simulink model "F16ASYM_Controlled_ACC"  (R2012b)
settings: Solver=ode3  SolverMode=SingleTasking  StartTime=0.0  StopTime=inf  FixedStep=T_sim  RelTol=1e-3
InitFcn:
  | load('NN_c_weights_Last_stable.mat')
values from neighbouring files (symbols this model uses):
  a1 = fitresult.p1    [Stall_protection.m]
  alpha_map_eval = ones(size(M_eval))*NaN    [Auto_trim_aid.m]    (also in Autotrim_maps.mat = [nan nan 0.277598136245 0.119432432992 0.0579479097061 0.027)
  beta_map_eval = ones(size(M_eval))*NaN    [Auto_trim_aid.m]    (also in Autotrim_maps.mat = [nan nan -0.00151549403324 0.00117807579006 -0.0052086799721)
  C_L_0 = fitresult.p2    [Stall_protection.m]
  G_eval = NaN*ones(size(M_sq,2),size(H_sq,2))    [Stall_protection.m]
  H_sq = unique(sort(H_sq))    [Stall_protection.m]
  H_sq_autotrim = min( F_envelope.H_1g):2000:max(F_envelope.H_1g)    [Auto_trim_aid.m]    (also in Autotrim_maps.mat = [0 2000 4000 6000 8000 10000 12000 14000 16000 18000])
  K_b_ACC = params(3)    [Cost_function.m]
  K_b_q = params(4)    [Cost_function.m]
  learning = 20    [Scheduling_desing.m]
  M_sq = unique(sort(M_sq))    [Stall_protection.m]
  M_sq_autotrim = 0:0.1:max(F_envelope.M_1g)    [Auto_trim_aid.m]    (also in Autotrim_maps.mat = [0 0.1 0.2 0.3 0.4 0.5 0.6 0.7 0.8 0.9 1 1.1 ... (21 element)
  Model_used_flag = 1    [Scheduling_desing.m]
  reg_param = 1    [Scheduling_desing.m]
  T_sim = 0.04    [Run_me.m]    (also in Scheduling_desing.m = 0.02)
  tau_ACC = params(1)    [Cost_function.m]
  tau_q = params(2)    [Cost_function.m]
  V_Comp_A_w_z_last = [-0.043311742939 0.0085685727899 -0.0213735657625 0.0330213821126 -0.0306555996667 -0.00573122365227 -0.0106441480787 0.0329440631876 0.0177121952361 -0.0290685435098 -0.0181457235686 -0.0361990502411 ... (1250 elements, 50x25)]    [NN_c_weights_Last_stable.mat]
  V_Comp_last = [-0.0421958473648 0.0184516098779 -0.0436695953504 -0.041154016657 0.00216882652165 -0.0388561228631 0.0327521861474 0.0326079628857 0.0227071838361 -0.0338588476214 0.0161615063846 0.00186003522421 ... (1250 elements, 50x25)]    [NN_c_weights_Last_stable.mat]
  velocity = M_eval(I,J)*a    [Auto_trim_aid.m]    (also in Scheduling_desing.m = M_eval_sche(I,J)*a)
  W_Comp_A_w_z_last = [-0.00689921461652 0.00234704735165 -0.000126421245896 0.00121944724496 6.17702028018e-05 -0.000422762754226 -0.000228913732743 -1.1618795843e-05 7.94007436465e-05 0.000588815786054 2.98617078429e-05 -0.00020420127191 ... (153 elements, 3x51)]    [NN_c_weights_Last_stable.mat]
  W_Comp_last = [-0.00864477030284 0.000183920433695 -0.000300268209456 0.00178165628538 -0.000144806488148 -0.000715209966 -0.000733452792184 5.9552378004e-05 0.000293789747621 0.00184648331608 -0.000150090451416 -0.000741280397229 ... (153 elements, 3x51)]    [NN_c_weights_Last_stable.mat]
undefined symbols (not defined in the file or in its folder): B, DiscIntNeverNeededParam, fi_flag_Simulink, k_B, m_B, sigbuilder_block, Stall_curve, Theta_1_roll_last, Theta_2_roll_last, Theta_3_roll_last, trim_control, trim_state, trim_throttle, V_long_lastA_w_z, V_long_lastAoA, V_roll_last, V_roll_lastMOD, V_yaw_last, W_long_lastA_w_z, W_long_lastAoA, W_roll_last, W_roll_lastMOD, W_yaw_last
libraries: Adaptive_FaultTolerantControl x43, F16_Actuator_Library x14, dspsigops x13, simulink x8, dsparch4 x6, simulink_extras x5, aerolibatmos2 x5, aerolibtransform2 x5, dspmtrx3 x3, qcatlib x2, dspvision x2, dspsnks4 x2
(part 3 of 10)

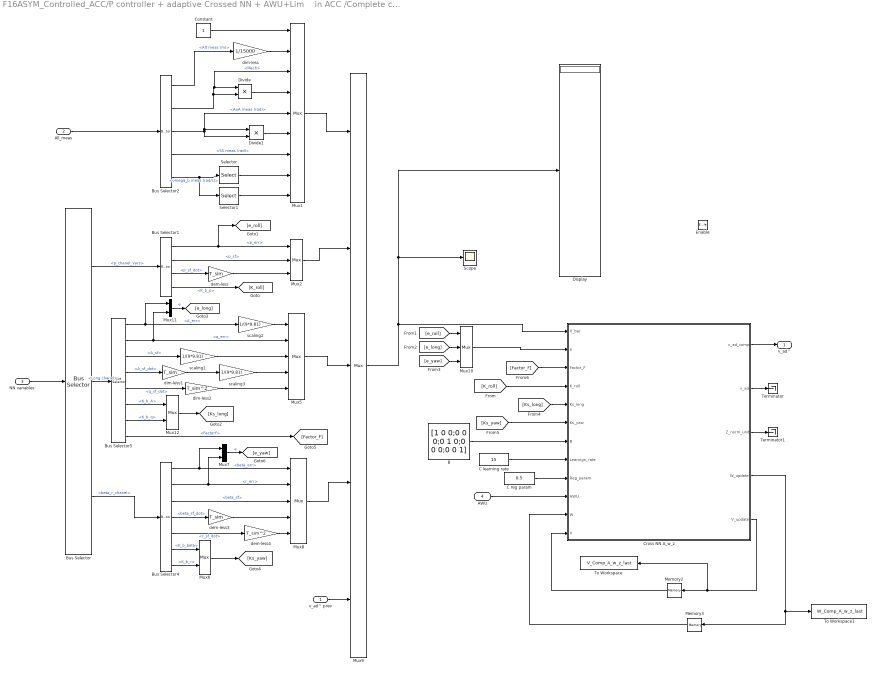
== system F16ASYM_Controlled_ACC/P controller + adaptive Crossed NN + AWU+Lim    in ACC /Complete crossed On-line (adaptive) multi-layer NN: A_w_z ==
  v_ad^ prev : Inport
  All_meas : Inport  Port=2
  NN variables : Inport  Port=3
  AWU : Inport  Port=4
  Enable : EnablePort  StatesWhenEnabling=reset
  B : Constant  Value=[1 0 0;0 0 0;0 1 0;0 0 0;0 0 1]
  Bus Selector : BusSelector  OutputSignals=p_chanel_vars,Long chanel,beta_r_chanel
  Bus Selector1 : BusSelector  OutputSignals=p_err,p_sf,p_sf_dot,K_b_p
  Bus Selector2 : BusSelector  OutputSignals=signal1.Alt meas (m),signal2.Mach,signal1.AoA meas (rad),signal1.SS meas (rad),signal1.omega_b meas (rad/s)
  Bus Selector4 : BusSelector  OutputSignals=beta_chanel vars.beta_err,r_chanel vars.r_err,beta_chanel vars.beta_sf,beta_chanel vars.beta_sf_dot,r_chanel vars.r_sf_dot,beta_chanel vars.K_b_beta,r_chanel vars.K_b_r
  Bus Selector5 : BusSelector  OutputSignals=A_chanel vars.A_err,q_chanel_vars.q_err,A_chanel vars.A_sf,A_chanel vars.A_sf_dot,q_chanel_vars.q_sf_dot,A_chanel vars.K_b_A,q_chanel_vars.K_b_q,A_chanel vars.FactorF
  C learning rate : Constant  Value=15  SampleTime=T_sim
  C reg param : Constant  Value=0.5  SampleTime=T_sim
  Constant : Constant
  Cross NN A_w_z : MATLAB Function  TreatAsAtomicUnit=on
  Display : Display
  Divide : Product  Inputs=**
  Divide1 : Product  Inputs=**
  Memory2 : Memory  X0=V_Comp_A_w_z_last
  Memory3 : Memory  X0=W_Comp_A_w_z_last
  Mux1 : Mux  Inputs=9
  Mux10 : Mux  Inputs=3
  Mux{6..7,11..12} (4 alike) : Mux  Inputs=2
  Mux2 : Mux  Inputs=3
  Mux5 : Mux  Inputs=5
  Mux8 : Mux  Inputs=5
  Mux9 : Mux  Inputs=[9 3 5 5 3]
  Scope : Scope
      settings: SaveName=ScopeData8
  Selector : Selector  InputPortWidth=3  IndexOptions=Index vector (dialog)  Indices=1  OutputSizes=1
  Selector1 : Selector  InputPortWidth=3  IndexOptions=Index vector (dialog)  Indices=3  OutputSizes=1
  Terminator : Terminator
  Terminator1 : Terminator
  To Workspace : ToWorkspace  VariableName=V_Comp_A_w_z_last  SampleTime=-1
      settings: MaxDataPoints=1
  To Workspace1 : ToWorkspace  VariableName=W_Comp_A_w_z_last  SampleTime=-1
      settings: MaxDataPoints=1
  dem-less : Gain  Gain=T_sim
  dem-less3 : Gain  Gain=T_sim
  dem-less4 : Gain  Gain=T_sim^2
  dim-less : Gain  Gain=1/15000
  dim-less1 : Gain  Gain=T_sim
  dim-less2 : Gain  Gain=T_sim^2
  scaling1 : Gain  Gain=1/(9*9.81)
  scaling2 : Gain  Gain=1/(9*9.81)
  scaling3 : Gain  Gain=1/(9*9.81)
  v_ad^ : Outport
  wires:
  [Factor_F] -> Cross NN A_w_z/3(Factor_F)
  Bus Selector5/8 -> [Factor_F]  "<FactorF>"
  scaling3/1 -> Mux5/4
  dim-less2/1 -> Mux5/5
  scaling1/1 -> Mux5/3
  Mux11/1 -> [e_long]  "e"
  Bus Selector/2 -> Bus Selector5/1  "<Long chanel>"
  Bus Selector5/1 -> Mux11/1, scaling2/1  "<A_err>"
  Bus Selector5/2 -> Mux11/2, Mux5/2  "<q_err>"
  Bus Selector5/3 -> scaling1/1  "<A_sf>"
  Bus Selector5/4 -> dim-less1/1  "<A_sf_dot>"
  Bus Selector5/5 -> dim-less2/1  "<q_sf_dot>"
  Bus Selector5/7 -> Mux12/2  "<K_b_q>"
  Bus Selector5/6 -> Mux12/1  "<K_b_A>"
  scaling2/1 -> Mux5/1
  dim-less1/1 -> scaling3/1
  Selector1/1 -> Mux1/9
  [Ks_yaw] -> Cross NN A_w_z/6(Ks_yaw)
  [Ks_long] -> Cross NN A_w_z/5(Ks_long)
  [K_roll] -> Cross NN A_w_z/4(K_roll)
  [e_yaw] -> Mux10/3
  [e_long] -> Mux10/2
  [e_roll] -> Mux10/1
  Mux10/1 -> Cross NN A_w_z/2(e)
  Cross NN A_w_z/4(W_update) -> To Workspace1/1, Memory3/1
  Cross NN A_w_z/5(V_update) -> Memory2/1, To Workspace/1
  Cross NN A_w_z/2(v_ad) -> Terminator/1
  B/1 -> Cross NN A_w_z/7(B)
  Memory3/1 -> Cross NN A_w_z/11(W)
  Memory2/1 -> Cross NN A_w_z/12(V)
  Cross NN A_w_z/1(v_ad_comp) -> v_ad^/1
  C learning rate/1 -> Cross NN A_w_z/8(Learnign_rate)
  C reg param/1 -> Cross NN A_w_z/9(Reg_param)
  Cross NN A_w_z/3(Z_norm_unit) -> Terminator1/1
  Mux9/1 -> Cross NN A_w_z/1(X_bar), Display/1, Scope/1
  v_ad^ prev/1 -> Mux9/5
  Mux8/1 -> Mux9/4
  Mux5/1 -> Mux9/3
  Mux2/1 -> Mux9/2
  Mux1/1 -> Mux9/1
  dem-less4/1 -> Mux8/5
  Mux7/1 -> [e_yaw]  "e"
  Bus Selector4/2 -> Mux7/2, Mux8/2  "<r_err>"
  Bus Selector4/1 -> Mux7/1, Mux8/1  "<beta_err>"
  Mux6/1 -> [Ks_yaw]
  Bus Selector4/6 -> Mux6/1  "<K_b_beta>"
  Bus Selector4/7 -> Mux6/2  "<K_b_r>"
  Bus Selector4/5 -> dem-less4/1  "<r_sf_dot>"
  Bus Selector4/4 -> dem-less3/1  "<beta_sf_dot>"
  Bus Selector4/3 -> Mux8/3  "<beta_sf>"
  dem-less3/1 -> Mux8/4
  Mux12/1 -> [Ks_long]
  dem-less/1 -> Mux2/3
  Bus Selector1/1 -> Mux2/1, [e_roll]  "<p_err>"
  Bus Selector1/2 -> Mux2/2  "<p_sf>"
  Bus Selector1/4 -> [K_roll]  "<K_b_p>"
  Bus Selector2/3 -> Divide1/2, Mux1/5, Divide1/1  "<AoA meas (rad)>"
  Bus Selector2/2 -> Divide/1, Mux1/3, Divide/2  "<Mach>"
  Bus Selector2/4 -> Mux1/7  "<SS meas (rad)>"
  Selector/1 -> Mux1/8
  Bus Selector1/3 -> dem-less/1  "<p_sf_dot>"
  Constant/1 -> Mux1/1
  All_meas/1 -> Bus Selector2/1
  Bus Selector2/1 -> dim-less/1  "<Alt meas (m)>"
  Divide/1 -> Mux1/4
  Divide1/1 -> Mux1/6
  dim-less/1 -> Mux1/2
  Bus Selector2/5 -> Selector/1, Selector1/1  "<omega_b meas (rad/s)>"
  NN variables/1 -> Bus Selector/1
  Bus Selector/1 -> Bus Selector1/1  "<p_chanel_vars>"
  Bus Selector/3 -> Bus Selector4/1  "<beta_r_chanel>"
  AWU/1 -> Cross NN A_w_z/10(AWU)

== system F16ASYM_Controlled_ACC/P controller + adaptive Crossed NN + AWU+Lim    in ACC /Lat_dir Dyn Inversion: beta_dot->r_c ==
  beta_dot_c : Inport
  All_meas : Inport  Port=2
  A_w_y : Selector  InputPortWidth=3  IndexOptions=Index vector (dialog)  Indices=2  OutputSizes=1
  Bus Selector : BusSelector  OutputSignals=signal1.AoA meas (rad),signal1.omega_b meas (rad/s),signal1.V_TAS (m/s),signal2.A_w_CG
  Divide1 : Product  Inputs=**
  Divide3 : Product  Inputs=**
  Divide4 : Product  Inputs=/*
  Divide5 : Product  Inputs=*/
  Selector : Selector  InputPortWidth=3  IndexOptions=Index vector (dialog)  Indices=1  OutputSizes=1
  Trigonometric Function : Trigonometry  Operator=cos
  Trigonometric Function3 : Trigonometry  Operator=tan
  "q_c " : Sum  Inputs=-++
  r_c : Outport
  wires:
  "q_c "/1 -> r_c/1
  Bus Selector/1 -> Trigonometric Function/1, Trigonometric Function3/1  "<AoA meas (rad)>"
  Bus Selector/2 -> Selector/1  "<omega_b meas (rad/s)>"
  Divide1/1 -> "q_c "/2
  Divide3/1 -> Divide4/1
  A_w_y/1 -> Divide4/2
  All_meas/1 -> Bus Selector/1
  Bus Selector/4 -> A_w_y/1  "<A_w_CG>"
  Divide4/1 -> "q_c "/3
  Bus Selector/3 -> Divide3/2  "<V_TAS (m/s)>"
  Trigonometric Function/1 -> Divide3/1, Divide5/2
  Divide5/1 -> "q_c "/1
  beta_dot_c/1 -> Divide5/1
  Trigonometric Function3/1 -> Divide1/1
  Selector/1 -> Divide1/2

== system F16ASYM_Controlled_ACC/P controller + adaptive Crossed NN + AWU+Lim    in ACC /Long Dyn Inversion: alpha_dot ->q ==
  alpha_dot_c : Inport
  All_meas : Inport  Port=2
  Completed : Subsystem
  Manual Switch : ManualSwitch
  Simplified : Subsystem
  q_c : Outport
  wires:
  alpha_dot_c/1 -> Simplified/1(alpha_dot_c), Completed/1(alpha_dot_c)
  All_meas/1 -> Simplified/2(All_meas), Completed/2(All_meas)
  Completed/1(q_c) -> Manual Switch/1
  Simplified/1(q_c) -> Manual Switch/2
  Manual Switch/1 -> q_c/1

== system F16ASYM_Controlled_ACC/P controller + adaptive Crossed NN + AWU+Lim    in ACC /Longitudinal controller in A_w_z ==
  A_w_z des : Inport
  AoA des (rad) : Inport  Port=2
  Anti-windup A_w_z : Inport  Port=3
  Anti-windup AoA : Inport  Port=4
  All meas : Inport  Port=5
  Accel rate --> AoA rate! : Subsystem
  Bus Creator : BusCreator  Inputs=5
  Bus Selector : BusSelector  OutputSignals=signal2.A_w_CG
  Divide : Product  Inputs=**
  Gain : Gain  Gain=-1
  Ref Model and P Controller : Subsystem
  Selector : Selector  InputPortWidth=3  IndexOptions=Index vector (dialog)  Indices=3  OutputSizes=1
  Stall protection : Subsystem  Commented=on
  Sum : Sum  Inputs=+-|
  Terminator : Terminator
  Terminator1 : Terminator
  Terminator2 : Terminator
  A_chanel vars : Outport
  alpha_dot_c : Outport  Port=2
  wires:
  Anti-windup AoA/1 -> Terminator1/1
  AoA des (rad)/1 -> Terminator/1
  Selector/1 -> Gain/1
  Gain/1 -> Ref Model and P Controller/2(y_meas)
  Bus Selector/1 -> Selector/1  "<A_w_CG>"
  Anti-windup A_w_z/1 -> Terminator2/1
  A_w_z des/1 -> Ref Model and P Controller/1(y_ref)
  Ref Model and P Controller/1(y_des_dot) -> Divide/1
  Ref Model and P Controller/2(y_c_ff_dot) -> Bus Creator/1  "A_sf_dot"
  Ref Model and P Controller/3(y_c) -> Bus Creator/2, Sum/1  "A_sf"
  Sum/1 -> Bus Creator/3  "A_err"
  Ref Model and P Controller/4(y_meas_out) -> Sum/2
  Ref Model and P Controller/5(k_b param) -> Bus Creator/4  "K_b_A"
  Bus Creator/1 -> A_chanel vars/1
  Divide/1 -> alpha_dot_c/1
  Accel rate --> AoA rate!/1(A_w  to AoA rates factor) -> Bus Creator/5, Divide/2  "FactorF"
  All meas/1 -> Bus Selector/1, Stall protection/2(All meas), Accel rate --> AoA rate!/1(All_meas)

== system F16ASYM_Controlled_ACC/P controller + adaptive Crossed NN + AWU+Lim    in ACC /Physical limitation ==
  note: Converto to Angular accelerations
  v comm : Inport
  all meas : Inport  Port=2
  Ang Accel : MATLAB Function
  Bus Selector : BusSelector  OutputSignals=signal1.Alt meas (m),signal1.V_TAS (m/s),signal1.AoA meas (rad),signal1.SS meas (rad),signal1.omega_b meas (rad/s),signal1.Throttle_meas
  Bus Selector1 : BusSelector  OutputSignals=signal2.q (Pa),signal1.omega_b meas (rad/s)
  Demux : Demux  Outputs=3
  Display : Display
  Display1 : Display
  Display2 : Display
  Divide : Product  Inputs=**
  Divide1 : Product  Inputs=**
  Gain : Gain  Gain=-1
  Gain1 : Gain
  Mom coefficients that was reached : MATLABFcn  MATLABFcn=Moms_Coeff_estimator  OutputDimensions=3  OutputSignalType=real
  Moments : Subsystem
  Mux : Mux  Inputs=3
  Mux1 : Mux  Inputs=7
  Saturation Dynamic : simulink/Discontinuities/Saturation Dynamic  OutMin=[]  OutMax=[]  OutDataTypeStr=Inherit: Same as second input  OutDataType=fixdt(1, 16)  OutScaling=2^-10  DoSatur=off
  Sign : Signum
  Sign1 : Signum
  max deflections estimator : MATLAB Function  TreatAsAtomicUnit=on
  v limted : Outport
  wires:
  max deflections estimator/1(max_defl) -> Mux1/7
  Mux1/1 -> Mom coefficients that was reached/1
  Bus Selector/5 -> Mux1/5  "<omega_b meas (rad/s)>"
  Bus Selector/1 -> Mux1/1  "<Alt meas (m)>"
  Bus Selector/2 -> Mux1/2  "<V_TAS (m/s)>"
  Bus Selector/3 -> Mux1/3  "<AoA meas (rad)>"
  Bus Selector/4 -> Mux1/4  "<SS meas (rad)>"
  Bus Selector/6 -> Mux1/6  "<Throttle_meas>"
  Ang Accel/2(q_dot) -> Mux/2
  Ang Accel/3(r_dot) -> Mux/3
  Ang Accel/1(p_dot) -> Mux/1
  Bus Selector1/2 -> Ang Accel/4(omega_b)  "<omega_b meas (rad/s)>"
  Moments/3(N) -> Ang Accel/3(N)
  Moments/2(M) -> Ang Accel/2(M)
  Moments/1(L) -> Ang Accel/1(L)
  Bus Selector1/1 -> Moments/4(q)  "<q (Pa)>"
  Demux/3 -> Moments/3(C_N)
  Demux/2 -> Moments/2(C_M)
  Demux/1 -> Moments/1(C_L)
  Mom coefficients that was reached/1 -> Demux/1
  all meas/1 -> Bus Selector/1, Bus Selector1/1
  Mux/1 -> Gain1/1
  v comm/1 -> Saturation Dynamic/2, Display1/1, max deflections estimator/1(v_comm)
  Saturation Dynamic/1 -> Display/1, v limted/1
  Sign/1 -> Divide/1
  Gain1/1 -> Divide/2, Divide1/1, Sign1/1, Display2/1, Sign/1
  Sign1/1 -> Gain/1
  Divide/1 -> Saturation Dynamic/1
  Gain/1 -> Divide1/2
  Divide1/1 -> Saturation Dynamic/3

== system F16ASYM_Controlled_ACC/P controller + adaptive Crossed NN + AWU+Lim    in ACC /Sigmoid  ==
  In : Inport
  Display : Display
  Fcn1 : Fcn  Commented=on  Expr=2.0 ./ (1.0 + exp(-u(4)*u(1:3)))-1
  MATLAB Function : MATLAB Function  TreatAsAtomicUnit=on
  a : Constant  Value=a
  Out : Outport
  wires:
  MATLAB Function/1(y) -> Display/1, Out/1
  In/1 -> MATLAB Function/1(u)
  a/1 -> MATLAB Function/2(a)

== matlab function F16ASYM_Controlled_ACC/Primary Controller/P controller + adaptive Isolated NN/On-line (adaptive) multi-layer NNs SIMPL/Roll NN/Roll 2HL NN/Roll Multilayer NN ==
  data: X_bar input size=[12,1]; v_ad_comp output; e input size=1; P input; B input; Roll_learnign_rate input size=1; Roll_reg_param input size=1; Theta_1 input size=[30,12]; Theta_2 input size=[20,31]; Theta_3 input size=[1,21]; v_ad output; Z_norm_unit output; T_sim parameter; Theta_1_update output; Theta_2_update output; Theta_3_update output
function [v_ad_comp,v_ad,Z_norm_unit,Theta_1_update,Theta_2_update,Theta_3_update]  = Roll_ML_NN(X_bar,e,P,B,Roll_learnign_rate, Roll_reg_param,Theta_1,Theta_2,Theta_3,T_sim)

%% Compute prelimiary parameters
zeta= e'*P*B;

%% Feedforward. Layers: Sigmoidal, linear, linear

a2=[1 ;  sigmoid( Theta_1*X_bar )]; % Sigmoidal
a3=[1 ;  (Theta_2*a2)]; % Linear
% z4=Theta_3*a3;
% a4 = z4; % Linear
% v_ad =a4;

% Backward
% % delta4=zeta; % In this particular case of adaptive NN, this error is a weighted tracking error
delta3=Theta_3'*zeta;
delta2=Theta_2'*delta3(2:end).*(a2.*(ones(size(a2))-a2)); 


%% Compute the gradients or adaptation laws
Gamma_Theta_3= Roll_learnign_rate; %  learnign rate
Gamma_Theta_2 = Roll_learnign_rate; % learning rate
Gamma_Theta_1= Roll_learnign_rate; % learning rate
lambda = Roll_reg_param;    % Regularization constant

% % Theta_1_dot=zeros(size(Theta_1));
% % Theta_2_dot=zeros(size(Theta_2));
% % Theta_3_dot=zeros(size(Theta_3));

Theta_3_dot = -Gamma_Theta_3*zeta*a3' ;
Theta_3_dot(:,2:end) =  Theta_3_dot(:,2:end) - Gamma_Theta_3*lambda*norm(zeta).*Theta_3(:,2:end);

Theta_2_dot= -Gamma_Theta_2*( delta3(2:end)*a2'   + lambda*norm(zeta).*Theta_2);
Theta_2_dot(:,2:end) =  Theta_2_dot(:,2:end) - Gamma_Theta_2*lambda*norm(zeta).*Theta_2(:,2:end);

Theta_1_dot= -Gamma_Theta_1*( delta2(2:end)*X_bar'   + lambda*norm(zeta).*Theta_1);
Theta_1_dot(:,2:end) =  Theta_1_dot(:,2:end) - Gamma_Theta_1*lambda*norm(zeta).*Theta_1(:,2:end);


%% Adaptation
Theta_1_update = Theta_1 + T_sim*Theta_1_dot;
Theta_2_update = Theta_2 + T_sim*Theta_2_dot;
Theta_3_update = Theta_3 + T_sim*Theta_3_dot;

%% re-compute v_ad

a2=[1 ;  sigmoid( Theta_1_update*X_bar )]; % Sigmoidal
a3=[1 ;  (Theta_2_update*a2)]; % Linear
v_ad=Theta_3_update*a3;


%% Compute v_ad_comp
% Z = blkdiag( Theta_1_update , Theta_2_update , Theta_3_update );

Z =  [ Theta_1_update, zeros(size(Theta_1_update,1),size(Theta_2_update,2)) , zeros(size(Theta_1_update,1),size(Theta_3_update,2));
            zeros(size(Theta_2_update,1),size(Theta_1_update,2)) , Theta_2_update , zeros(size(Theta_2_update,1),size(Theta_3_update,2)) ;
            zeros(size(Theta_3_update,1),size(Theta_1_update,2)),zeros(size(Theta_3_update,1),size(Theta_2_update,2)),  Theta_3_update ];

Z_norm = norm(Z,'fro');
Z_max = min(size(Theta_1))*min(size(Theta_2))*min(size(Theta_3));
Z_norm_unit = Z_norm;

K_r0= 0.02;
K_r1= 0;
v_r0 = -K_r0*zeta;
v_r1 = -K_r1*(Z_norm+Z_max)*zeta;

v_ad_comp = v_ad + v_r1 +v_r0;


end

== matlab function F16ASYM_Controlled_ACC/Control allocator/Control allocator: NO RECONF/MATLAB Function ==
  data: Deflections input; Saturations output; Sup_lim input; Inf_lim input
function Saturations = Saturations(Deflections,Sup_lim,Inf_lim)
Saturations=zeros(7,1);

for i=1:7
    
    if Deflections(i)>=Sup_lim(i)
        Saturations(i)=1;
    elseif Deflections(i)<=Inf_lim(i)
        Saturations(i)=-1;
    else
        Saturations(i)=0;
    end
end

== matlab function F16ASYM_Controlled_ACC/Anti-windup Calculation/Anti-windup: Reconfigurable/Antiwindup calculation ==
  data: Ang_acell_comm input; AWU output; Ang_acell_achieved input; Saturations input; B input; deflections input
function AWU = AWU_calculation(Ang_acell_comm,Ang_acell_achieved,Saturations,B,deflections)
% Computing Saturation limits
sup_limit = [24,24,21,21,29,25,25]-1;
inf_limit = [-24,-24,-21,-21,-29,0,0]+1;

for i=1:7
    Saturations(i) = Saturation_smooth(abs(Saturations(i)),deflections(i),sup_limit(i),inf_limit(i));
end
Sat_B = B*Saturations;
B_max = B*ones(7,1);

AWU=zeros(3,1);

%% Method A
% % psi = 0.01; % % of the effort above the one we consider manouvreability is reduced
% % for i=1:3
% %     if i==1 && sign(deflections(3))== sign(deflections(4)) && abs(Sat_B(i))>psi*abs(B_max(i))
% %         AWU(2) = Ang_acell_comm(2) - Ang_acell_achieved(2); % we have to desaturate longitudinally not laterally
% %     elseif  i==1 && sign(deflections(3))~= sign(deflections(4)) && abs(Sat_B(i))>psi*abs(B_max(i))
% %         AWU(i) = Ang_acell_comm(i) - Ang_acell_achieved(i);
% %     elseif i~=1 && abs(Sat_B(i))>psi*abs(B_max(i))
% %         AWU(i) = Ang_acell_comm(i) - Ang_acell_achieved(i);
% %     end 
% % end

%% Method B
% % % Long
% % if Saturations(1)~=0 || Saturations(2)~=0 ||  Saturations(6)~=0 || Saturations(7)~=0 || ((Saturations(3)~=0 || Saturations(4)~=0) && sign(deflections(3))== sign(deflections(4)) ) 
% %     AWU(2) = Ang_acell_comm(2) - Ang_acell_achieved(2);
% % end
% % % Lat-dir
% % if ((Saturations(3)~=0 || Saturations(4)~=0) && sign(deflections(3)) ~= sign(deflections(4)) )  || Saturations(5)~=0 || Saturations(6)~=0 || Saturations(7)~=0
% %     AWU(1) = Ang_acell_comm(1) - Ang_acell_achieved(1);
% %     AWU(3) = Ang_acell_comm(3) - Ang_acell_achieved(3);
% % 
% % end


%% Method C
for i=1:3
        AWU(i) = (Ang_acell_comm(i) - Ang_acell_achieved(i))*Sat_B(i)/norm(B(i,:));
end

end

function Saturation_out = Saturation_smooth(Saturation,angle,sup_limit,inf_limit)

a=5;
Saturation_out  = ( 1 - 1./(1+exp(-a*(angle-inf_limit ))) + 1./(1+exp(-a*(angle-sup_limit ))) )*Saturation;


end

== matlab function F16ASYM_Controlled_ACC/Primary Controller/P  + Crossed NN + AWU+Lim + hand-over/P controller + adaptive Crossed NN + AWU+Lim   in AoA/Physical limitation/Ang Accel ==
  data: L input; p_dot output; q_dot output; r_dot output; M input; N input; omega_b input
function [p_dot,q_dot,r_dot] = Ang_accel(L,M,N,omega_b)
Jy  = 75673.6;
Jxz = 1331.4; 
Jz  = 85552.1;  
Jx  = 12874.8;
h_E = 216.9;

denom = Jx*Jz - Jxz*Jxz;

% % C1 = ((Jy - Jz)  * Jz  - (Jxz * Jxz))/ Gamma;
% % C2 = ((Jx - Jy + Jz ) * Jxz ) / Gamma;
% % C3 = Jz / Gamma;
% % C4 = Jxz / Gamma;
% % C5 = (Jz - Jx) / Jy;
% % C6 = Jxz / Jy ;
% % C7 = 1 / Jy;
% % C8 = (Jx * (Jx - Jy ) + Jxz * Jxz) / Gamma;
% % C9 = Jx / Gamma;


p_dot =  (Jz*L + Jxz*N - (Jz*(Jz-Jy)+Jxz*Jxz)*omega_b(2)*omega_b(3) + Jxz*(Jx-Jy+Jz)*omega_b(1)*omega_b(2) + Jxz*omega_b(2)*h_E)/denom;

q_dot = (M + (Jz-Jx)*omega_b(1)*omega_b(3) - Jxz*(omega_b(1)*omega_b(1)-omega_b(3)*omega_b(3)) - omega_b(3)*h_E)/Jy;


r_dot = (Jx*N + Jxz*L + (Jx*(Jx-Jy)+Jxz*Jxz)*omega_b(1)*omega_b(2) - Jxz*(Jx-Jy+Jz)*omega_b(2)*omega_b(3) +  Jx*omega_b(2)*h_E)/denom;

== matlab function F16ASYM_Controlled_ACC/P controller + adaptive Crossed NN + AWU+Lim    in ACC /Physical limitation/Ang Accel ==
  data: L input; p_dot output; q_dot output; r_dot output; M input; N input; omega_b input
function [p_dot,q_dot,r_dot] = Ang_accel(L,M,N,omega_b)
Jy  = 75673.6;
Jxz = 1331.4; 
Jz  = 85552.1;  
Jx  = 12874.8;
h_E = 216.9;

denom = Jx*Jz - Jxz*Jxz;

% % C1 = ((Jy - Jz)  * Jz  - (Jxz * Jxz))/ Gamma;
% % C2 = ((Jx - Jy + Jz ) * Jxz ) / Gamma;
% % C3 = Jz / Gamma;
% % C4 = Jxz / Gamma;
% % C5 = (Jz - Jx) / Jy;
% % C6 = Jxz / Jy ;
% % C7 = 1 / Jy;
% % C8 = (Jx * (Jx - Jy ) + Jxz * Jxz) / Gamma;
% % C9 = Jx / Gamma;


p_dot =  (Jz*L + Jxz*N - (Jz*(Jz-Jy)+Jxz*Jxz)*omega_b(2)*omega_b(3) + Jxz*(Jx-Jy+Jz)*omega_b(1)*omega_b(2) + Jxz*omega_b(2)*h_E)/denom;

q_dot = (M + (Jz-Jx)*omega_b(1)*omega_b(3) - Jxz*(omega_b(1)*omega_b(1)-omega_b(3)*omega_b(3)) - omega_b(3)*h_E)/Jy;


r_dot = (Jx*N + Jxz*L + (Jx*(Jx-Jy)+Jxz*Jxz)*omega_b(1)*omega_b(2) - Jxz*(Jx-Jy+Jz)*omega_b(2)*omega_b(3) +  Jx*omega_b(2)*h_E)/denom;

== system F16ASYM_Controlled_ACC/Primary Controller/P  + Crossed NN + AWU+Lim + hand-over ==
  note: Indicator correspond to 1
  note: Indicator correspond to 0
  A_w_z des : Inport
  AoA des (rad) : Inport  Port=2
  p des (rad/s) : Inport  Port=3
  beta des (rad) : Inport  Port=4
  Anti-windup A_w_z : Inport  Port=5
  Anti-windup AoA : Inport  Port=6
  Anti-windup beta : Inport  Port=7
  All measures : Inport  Port=8
  Anti-windup signals : Inport  Port=9
  A_w_z des1 : InportShadow
  Anti-windup A_w_z1 : InportShadow  Port=5
  Anti-windup AoA1 : InportShadow  Port=6
  Anti-windup beta1 : InportShadow  Port=7
  Anti-windup signals1 : InportShadow  Port=9
  AoA des (rad)1 : InportShadow  Port=2
  Bus Selector : BusSelector  OutputSignals=signal2.a,signal1.V_TAS (m/s)
  Gain2 : Gain  Gain=2
  Logical Operator : Logic  Operator=NOT  AllPortsSameDT=off  OutDataTypeStr=boolean
  Min TAS : Product  Inputs=**
  "P controller + adaptive Crossed NN + AWU+Lim    in ACC " : Subsystem  VariantObject=Adaptive Controller Crossed+AWU+Lim
  P controller + adaptive Crossed NN + AWU+Lim   in AoA : Subsystem  VariantObject=Adaptive Controller Crossed+AWU+Lim
  Relational Operator5 : RelationalOperator  OutDataTypeStr=boolean
  Scope : Scope
      settings: YMin=-2.75  YMax=0.25  SaveName=ScopeData32
  Scope1 : Scope  Commented=on
      settings: YMin=-2.75  YMax=0.25  SaveName=ScopeData33
  Switch : Switch  Commented=on  Threshold=0.5  InputSameDT=on
  Transition smoother : MATLAB Function  Commented=on  TreatAsAtomicUnit=on
  "Transitions Smotother " : Subsystem
  Transitions Smotother 1 : Subsystem  Commented=on
  Unit Delay : UnitDelay  Commented=on  SampleTime=-1
  beta des (rad)1 : InportShadow  Port=4
  p des (rad/s)1 : InportShadow  Port=3
  Angular acc des : Outport
  Control_in : Outport  Port=2
  wires:
  Anti-windup signals/1 -> P controller + adaptive Crossed NN + AWU+Lim   in AoA/9(Anti-windup signals)
  Anti-windup beta/1 -> P controller + adaptive Crossed NN + AWU+Lim   in AoA/7(Anti-windup beta)
  A_w_z des/1 -> P controller + adaptive Crossed NN + AWU+Lim   in AoA/1(A_w_z des)
  Anti-windup A_w_z/1 -> P controller + adaptive Crossed NN + AWU+Lim   in AoA/5(Anti-windup A_w_z)
  Anti-windup AoA/1 -> P controller + adaptive Crossed NN + AWU+Lim   in AoA/6(Anti-windup AoA)
  AoA des (rad)/1 -> P controller + adaptive Crossed NN + AWU+Lim   in AoA/2(AoA des (rad))
  beta des (rad)/1 -> P controller + adaptive Crossed NN + AWU+Lim   in AoA/4(beta des (rad))
  p des (rad/s)/1 -> P controller + adaptive Crossed NN + AWU+Lim   in AoA/3(p des (rad/s))
  A_w_z des1/1 -> "P controller + adaptive Crossed NN + AWU+Lim    in ACC "/1(A_w_z des)
  AoA des (rad)1/1 -> "P controller + adaptive Crossed NN + AWU+Lim    in ACC "/2(AoA des (rad))
  p des (rad/s)1/1 -> "P controller + adaptive Crossed NN + AWU+Lim    in ACC "/3(p des (rad/s))
  beta des (rad)1/1 -> "P controller + adaptive Crossed NN + AWU+Lim    in ACC "/4(beta des (rad))
  Anti-windup A_w_z1/1 -> "P controller + adaptive Crossed NN + AWU+Lim    in ACC "/5(Anti-windup A_w_z)
  Anti-windup AoA1/1 -> "P controller + adaptive Crossed NN + AWU+Lim    in ACC "/6(Anti-windup AoA)
  Anti-windup beta1/1 -> "P controller + adaptive Crossed NN + AWU+Lim    in ACC "/7(Anti-windup beta)
  All measures/1 -> "P controller + adaptive Crossed NN + AWU+Lim    in ACC "/8(All measures), Bus Selector/1, P controller + adaptive Crossed NN + AWU+Lim   in AoA/8(All measures)
  Anti-windup signals1/1 -> "P controller + adaptive Crossed NN + AWU+Lim    in ACC "/9(Anti-windup signals)
  [Min_Mach] -> Min TAS/1  "Min M"
  Bus Selector/1 -> Min TAS/2  "<a>"
  Min TAS/1 -> Gain2/1
  Gain2/1 -> Relational Operator5/1
  Bus Selector/2 -> Relational Operator5/2  "<V_TAS (m/s)>"
  "P controller + adaptive Crossed NN + AWU+Lim    in ACC "/1(Angular acc des) -> "Transitions Smotother "/3(From  ACC)
  P controller + adaptive Crossed NN + AWU+Lim   in AoA/1(Angular acc des) -> "Transitions Smotother "/1(From AoA)
  Relational Operator5/1 -> Logical Operator/1, Control_in/1, "Transitions Smotother "/2(Indicator), P controller + adaptive Crossed NN + AWU+Lim   in AoA/10(Active)
  Transition smoother/2(indicator_out) -> Unit Delay/1
  Unit Delay/1 -> Transition smoother/4(indicator_prev)
  "Transitions Smotother "/1(Ang accels comm) -> Angular acc des/1, Scope/1
  Switch/1 -> Scope1/1
  Logical Operator/1 -> "P controller + adaptive Crossed NN + AWU+Lim    in ACC "/10(Active)

== system F16ASYM_Controlled_ACC/Primary Controller/P controller ==
  A_w_z des : Inport
  AoA des (rad) : Inport  Port=2
  p des (rad/s) : Inport  Port=3
  beta des (rad) : Inport  Port=4
  Anti-windup A_w_z : Inport  Port=5
  Anti-windup AoA : Inport  Port=6
  Anti-windup beta : Inport  Port=7
  All measures : Inport  Port=8
  Anti-windup signals : Inport  Port=9
  Body Rates Controller : Subsystem
  Bus Creator2 : BusCreator
  Bus Selector3 : BusSelector  OutputSignals=signal1.SS meas (rad)
  Constant : Constant  Value=NaN
  Display : Display
  Display1 : Display
  Lat_dir Dyn Inversion: beta_dot->r_c : Subsystem
  Long Dyn Inversion: alpha_dot ->q : Subsystem
  Longitudinal Controller: AoA or A_w_z : Subsystem  Variant=on  OverrideUsingVariant=Controller of AoA
  Ref Model and P Controller : Adaptive_FaultTolerantControl/Ref Model and P Controller  tau=0.4  y_i=trim_state(9)  K_f=1  K_b=5
  Sum1 : Sum  Inputs=+-|
  Terminator : Terminator
  Terminator1 : Terminator
  Terminator2 : Terminator
  Angular acc des : Outport
  Control_in : Outport  Port=2
  wires:
  Anti-windup beta/1 -> Terminator1/1
  Ref Model and P Controller/5 -> Bus Creator2/4  "K_b_beta"
  Ref Model and P Controller/4 -> Sum1/2
  Sum1/1 -> Bus Creator2/3  "beta_err"
  Ref Model and P Controller/3 -> Bus Creator2/2, Sum1/1  "beta_sf"
  Ref Model and P Controller/2 -> Bus Creator2/1  "beta_sf_dot"
  Anti-windup signals/1 -> Terminator/1
  All measures/1 -> Longitudinal Controller: AoA or A_w_z/5(All meas), Long Dyn Inversion: alpha_dot ->q/2(All_meas), Bus Selector3/1, Lat_dir Dyn Inversion: beta_dot->r_c/2(All_meas), Body Rates Controller/4(All_meas)
  A_w_z des/1 -> Longitudinal Controller: AoA or A_w_z/1(A_w_z des)
  Anti-windup A_w_z/1 -> Longitudinal Controller: AoA or A_w_z/3(Anti-windup A_w_z)
  Anti-windup AoA/1 -> Longitudinal Controller: AoA or A_w_z/4(Anti-windup AoA)
  AoA des (rad)/1 -> Longitudinal Controller: AoA or A_w_z/2(AoA des (rad))
  Longitudinal Controller: AoA or A_w_z/3(alpha_dot_c) -> Display/1, Long Dyn Inversion: alpha_dot ->q/1(alpha_dot_c)
  beta des (rad)/1 -> Ref Model and P Controller/1
  Long Dyn Inversion: alpha_dot ->q/1(q_c) -> Body Rates Controller/2(q_ref), Display1/1
  p des (rad/s)/1 -> Body Rates Controller/1(p_ref)
  Ref Model and P Controller/1 -> Lat_dir Dyn Inversion: beta_dot->r_c/1(beta_dot_c)
  Bus Selector3/1 -> Ref Model and P Controller/2  "<SS meas (rad)>"
  Lat_dir Dyn Inversion: beta_dot->r_c/1(r_c) -> Body Rates Controller/3(r_ref)
  Bus Creator2/1 -> Terminator2/1  "beta_chanel vars"
  Body Rates Controller/1(Angular acc des (rad/s^2)) -> Angular acc des/1  "v_p+v_dot_ff"
  Constant/1 -> Control_in/1

== system F16ASYM_Controlled_ACC/Primary Controller/P controller + adaptive Crossed NN ==
  A_w_z des : Inport
  AoA des (rad) : Inport  Port=2
  p des (rad/s) : Inport  Port=3
  beta des (rad) : Inport  Port=4
  Anti-windup A_w_z : Inport  Port=5
  Anti-windup AoA : Inport  Port=6
  Anti-windup beta : Inport  Port=7
  All measures : Inport  Port=8
  Anti-windup signals : Inport  Port=9
  Body Rates Controller : Subsystem
  Bus Creator : BusCreator  Inputs=3
  Bus Creator1 : BusCreator  Inputs=3
  Bus Creator2 : BusCreator
  Bus Creator3 : BusCreator  Inputs=2
  Bus Selector3 : BusSelector  OutputSignals=signal1.SS meas (rad)
  Complete crossed On-line (adaptive) multi-layer NN : Subsystem  Variant=on  OverrideUsingVariant=NN on A_w_z
      mask Display:
      | image(imread('ANN.png'))
      | 
      | port_label('input', 1, 'v prev')
      | port_label('input', 2, 'All meas')
      | port_label('input', 3, 'NN vars')
      | 
      | port_label('output', 1, 'v_ad^')
  Display{,1..6} (7 alike) : Display
  Ground : Ground
  Lat_dir Dyn Inversion: beta_dot->r_c : Subsystem
  Long Dyn Inversion: alpha_dot ->q : Subsystem
  Longitudinal Controller: AoA or A_w_z : Subsystem  Variant=on  OverrideUsingVariant=Controller of A_w_z
  Memory : Memory  X0=[0,0,0]
  Ref Model and P Controller : Adaptive_FaultTolerantControl/Ref Model and P Controller  tau=0.45  y_i=trim_state(9)  K_f=1  K_b=5
  "Sigmoid " : Subsystem  mask{a=0.15}
      mask prompts: a "Sigmoid a param"
      mask TypeOptions a: a/Value
      mask Display:
      | x=-25:0.1:25;
      | 
      | y=(2.0 ./ (1.0 + exp(-a.*x))-1) ;
      | y2=zeros(size(x));
      | 
      | plot(x,y,x,y2);
      | 
      | text(-12,0.5, ['a= ',num2str(a)])
  Sum : Sum  Inputs=-+|
  Sum1 : Sum  Inputs=+-|
  Terminator : Terminator
  Terminator1 : Terminator
  Angular acc des : Outport
  Control_in : Outport  Port=2
  wires:
  Anti-windup signals/1 -> Terminator/1
  Ref Model and P Controller/1 -> Lat_dir Dyn Inversion: beta_dot->r_c/1(beta_dot_c), Display5/1
  Complete crossed On-line (adaptive) multi-layer NN/1(v_ad^) -> Display2/1, Sum/1  "v_ad^"
  "Sigmoid "/1(Out) -> Memory/1
  Anti-windup beta/1 -> Terminator1/1
  Bus Creator3/1 -> Bus Creator/3  "beta_r_chanel"
  Bus Creator2/1 -> Bus Creator3/2  "beta_chanel vars"
  Body Rates Controller/3(r_chanel vars) -> Bus Creator3/1  "r_chanel vars"
  Ref Model and P Controller/5 -> Bus Creator2/4  "K_b_beta"
  Ref Model and P Controller/4 -> Sum1/2
  Sum1/1 -> Bus Creator2/3  "beta_err"
  Ref Model and P Controller/3 -> Bus Creator2/2, Sum1/1  "beta_sf"
  Ref Model and P Controller/2 -> Bus Creator2/1  "beta_sf_dot"
  Bus Creator1/1 -> Bus Creator/1  "Long chanel"
  Longitudinal Controller: AoA or A_w_z/2(alpha_chanel vars) -> Bus Creator1/2  "alpha_chanel vars"
  Longitudinal Controller: AoA or A_w_z/1(A_chanel vars) -> Bus Creator1/1  "A_chanel vars"
  Body Rates Controller/1(q_chanel vars) -> Bus Creator1/3  "q_chanel_vars"
  Body Rates Controller/2(p_chanel vars) -> Bus Creator/2  "p_chanel_vars"
  Memory/1 -> Complete crossed On-line (adaptive) multi-layer NN/1(v_ad^ prev)
  Bus Creator/1 -> Complete crossed On-line (adaptive) multi-layer NN/3(NN variables)
  Body Rates Controller/4(Angular acc des (rad/s^2)) -> Sum/2, Display3/1  "v_p+v_dot_ff"
  All measures/1 -> Longitudinal Controller: AoA or A_w_z/5(All meas), Long Dyn Inversion: alpha_dot ->q/2(All_meas), Bus Selector3/1, Lat_dir Dyn Inversion: beta_dot->r_c/2(All_meas), Body Rates Controller/4(All_meas), Complete crossed On-line (adaptive) multi-layer NN/2(All_meas)
  Sum/1 -> Angular acc des/1, "Sigmoid "/1(In), Display4/1  "v"
  A_w_z des/1 -> Longitudinal Controller: AoA or A_w_z/1(A_w_z des)
  Anti-windup A_w_z/1 -> Longitudinal Controller: AoA or A_w_z/3(Anti-windup A_w_z)
  Anti-windup AoA/1 -> Longitudinal Controller: AoA or A_w_z/4(Anti-windup AoA)
  AoA des (rad)/1 -> Longitudinal Controller: AoA or A_w_z/2(AoA des (rad))
  Longitudinal Controller: AoA or A_w_z/3(alpha_dot_c) -> Display/1, Long Dyn Inversion: alpha_dot ->q/1(alpha_dot_c)
  beta des (rad)/1 -> Ref Model and P Controller/1
  Long Dyn Inversion: alpha_dot ->q/1(q_c) -> Body Rates Controller/2(q_ref), Display1/1
  p des (rad/s)/1 -> Body Rates Controller/1(p_ref)
  Bus Selector3/1 -> Ref Model and P Controller/2  "<SS meas (rad)>"
  Lat_dir Dyn Inversion: beta_dot->r_c/1(r_c) -> Body Rates Controller/3(r_ref), Display6/1
  Ground/1 -> Control_in/1

== system F16ASYM_Controlled_ACC/Primary Controller/P controller + adaptive Crossed NN + AWU+Lim  ==
  A_w_z des : Inport
  AoA des (rad) : Inport  Port=2
  p des (rad/s) : Inport  Port=3
  beta des (rad) : Inport  Port=4
  Anti-windup A_w_z : Inport  Port=5
  Anti-windup AoA : Inport  Port=6
  Anti-windup beta : Inport  Port=7
  All measures : Inport  Port=8
  Anti-windup signals : Inport  Port=9
  Body Rates Controller : Subsystem
  Bus Creator : BusCreator  Inputs=3
  Bus Creator1 : BusCreator  Inputs=3
  Bus Creator2 : BusCreator
  Bus Creator3 : BusCreator  Inputs=2
  Bus Selector3 : BusSelector  OutputSignals=signal1.SS meas (rad)
  Complete crossed On-line (adaptive) multi-layer NN : Subsystem  Variant=on  OverrideUsingVariant=NN on AoA
      mask Display:
      | image(imread('ANN.png'))
      | 
      | port_label('input', 1, 'v prev')
      | port_label('input', 2, 'All meas')
      | port_label('input', 3, 'NN vars')
      | port_label('input', 4, 'Anti-windup')
      | 
      | port_label('output', 1, 'v_ad^')
  Constant : Constant  Value=NaN
  Display{,1..3,5..6} (6 alike) : Display
  "Display4 " : Display
  Lat_dir Dyn Inversion: beta_dot->r_c : Subsystem
  Long Dyn Inversion: alpha_dot ->q : Subsystem
  Longitudinal Controller: AoA or A_w_z : Subsystem  Variant=on  OverrideUsingVariant=Controller of AoA
  Memory : Memory  X0=[0,0,0]
  Physical limitation : Subsystem
  Ref Model and P Controller : Adaptive_FaultTolerantControl/Ref Model and P Controller  tau=0.45  y_i=trim_state(9)  K_f=1  K_b=5
  Scope1 : Scope
      settings: YMin=-8000  YMax=9000  SaveName=ScopeData27
  "Sigmoid " : Subsystem  mask{a=0.15}
      mask prompts: a "Sigmoid a param"
      mask TypeOptions a: a/Value
      mask Display:
      | x=-25:0.1:25;
      | 
      | y=(2.0 ./ (1.0 + exp(-a.*x))-1) ;
      | y2=zeros(size(x));
      | 
      | plot(x,y,x,y2);
      | 
      | text(-12,0.5, ['a= ',num2str(a)])
  Sum : Sum  Inputs=-+|
  Sum1 : Sum  Inputs=+-|
  Terminator1 : Terminator
  Angular acc des : Outport
  Control_in : Outport  Port=2
  wires:
  Lat_dir Dyn Inversion: beta_dot->r_c/1(r_c) -> Display6/1, Body Rates Controller/3(r_ref)
  Bus Selector3/1 -> Ref Model and P Controller/2  "<SS meas (rad)>"
  p des (rad/s)/1 -> Body Rates Controller/1(p_ref)
  Long Dyn Inversion: alpha_dot ->q/1(q_c) -> Body Rates Controller/2(q_ref), Display1/1
  beta des (rad)/1 -> Ref Model and P Controller/1
  Longitudinal Controller: AoA or A_w_z/3(alpha_dot_c) -> Long Dyn Inversion: alpha_dot ->q/1(alpha_dot_c), Display/1
  AoA des (rad)/1 -> Longitudinal Controller: AoA or A_w_z/2(AoA des (rad))
  Anti-windup AoA/1 -> Longitudinal Controller: AoA or A_w_z/4(Anti-windup AoA)
  Anti-windup A_w_z/1 -> Longitudinal Controller: AoA or A_w_z/3(Anti-windup A_w_z)
  A_w_z des/1 -> Longitudinal Controller: AoA or A_w_z/1(A_w_z des)
  Sum/1 -> "Display4 "/1, "Sigmoid "/1(In), Physical limitation/1(v comm)  "v"
  All measures/1 -> Complete crossed On-line (adaptive) multi-layer NN/2(All_meas), Physical limitation/2(all meas), Body Rates Controller/4(All_meas), Lat_dir Dyn Inversion: beta_dot->r_c/2(All_meas), Bus Selector3/1, Long Dyn Inversion: alpha_dot ->q/2(All_meas), Longitudinal Controller: AoA or A_w_z/5(All meas)
  Body Rates Controller/4(Angular acc des (rad/s^2)) -> Display3/1, Sum/2  "v_p+v_dot_ff"
  Bus Creator/1 -> Complete crossed On-line (adaptive) multi-layer NN/3(NN variables)
  Memory/1 -> Complete crossed On-line (adaptive) multi-layer NN/1(v_ad^ prev)
  Body Rates Controller/2(p_chanel vars) -> Bus Creator/2  "p_chanel_vars"
  Body Rates Controller/1(q_chanel vars) -> Bus Creator1/3  "q_chanel_vars"
  Longitudinal Controller: AoA or A_w_z/1(A_chanel vars) -> Bus Creator1/1  "A_chanel vars"
  Longitudinal Controller: AoA or A_w_z/2(alpha_chanel vars) -> Bus Creator1/2  "alpha_chanel vars"
  Bus Creator1/1 -> Bus Creator/1  "Long chanel"
  Ref Model and P Controller/2 -> Bus Creator2/1  "beta_sf_dot"
  Ref Model and P Controller/3 -> Sum1/1, Bus Creator2/2  "beta_sf"
  Sum1/1 -> Bus Creator2/3  "beta_err"
  Ref Model and P Controller/4 -> Sum1/2
  Ref Model and P Controller/5 -> Bus Creator2/4  "K_b_beta"
  Body Rates Controller/3(r_chanel vars) -> Bus Creator3/1  "r_chanel vars"
  Bus Creator2/1 -> Bus Creator3/2  "beta_chanel vars"
  Bus Creator3/1 -> Bus Creator/3  "beta_r_chanel"
  Anti-windup beta/1 -> Terminator1/1
  "Sigmoid "/1(Out) -> Memory/1
  Complete crossed On-line (adaptive) multi-layer NN/1(v_ad^) -> Scope1/1, Display2/1, Sum/1  "v_ad^"
  Ref Model and P Controller/1 -> Display5/1, Lat_dir Dyn Inversion: beta_dot->r_c/1(beta_dot_c)
  Anti-windup signals/1 -> Complete crossed On-line (adaptive) multi-layer NN/4(AWU)
  Physical limitation/1(v limted) -> Angular acc des/1
  Constant/1 -> Control_in/1

== system F16ASYM_Controlled_ACC/Primary Controller/P controller + adaptive Isolated NN ==
  A_w_z des : Inport
  AoA des (rad) : Inport  Port=2
  p des (rad/s) : Inport  Port=3
  beta des (rad) : Inport  Port=4
  Anti-windup A_w_z : Inport  Port=5
  Anti-windup AoA : Inport  Port=6
  Anti-windup beta : Inport  Port=7
  All measures : Inport  Port=8
  Anti-windup signals : Inport  Port=9
  Body Rates Controller : Subsystem
  Bus Creator : BusCreator  Inputs=3
  Bus Creator1 : BusCreator  Inputs=3
  Bus Creator2 : BusCreator
  Bus Creator3 : BusCreator  Inputs=2
  Bus Selector3 : BusSelector  OutputSignals=signal1.SS meas (rad)
  Display{,1..6} (7 alike) : Display
  Ground : Ground
  Lat_dir Dyn Inversion: beta_dot->r_c : Subsystem
  Long Dyn Inversion: alpha_dot ->q : Subsystem
  Longitudinal Controller: AoA or A_w_z : Subsystem  Variant=on  OverrideUsingVariant=Controller of A_w_z
  Memory : Memory  X0=[0,0,0]
  On-line (adaptive) multi-layer NNs : Subsystem
      mask Display:
      | image(imread('ANN.png'))
      | 
      | port_label('input', 1, 'v prev')
      | port_label('input', 2, 'All meas')
      | port_label('input', 3, 'NN vars')
      | 
      | port_label('output', 1, 'v_ad^')
  On-line (adaptive) multi-layer NNs SIMPL : Subsystem  Commented=on
      mask Display:
      | image(imread('ANN.png'))
      | 
      | port_label('input', 1, 'v prev')
      | port_label('input', 2, 'All meas')
      | port_label('input', 3, 'NN vars')
      | 
      | port_label('output', 1, 'v_ad^')
  Ref Model and P Controller : Adaptive_FaultTolerantControl/Ref Model and P Controller  tau=0.45  y_i=trim_state(9)  K_f=1  K_b=5
  "Sigmoid " : Subsystem  mask{a=0.15}
      mask prompts: a "Sigmoid a param"
      mask TypeOptions a: a/Value
      mask Display:
      | x=-25:0.1:25;
      | 
      | y=(2.0 ./ (1.0 + exp(-a.*x))-1) ;
      | y2=zeros(size(x));
      | 
      | plot(x,y,x,y2);
      | 
      | text(-12,0.5, ['a= ',num2str(a)])
  Sum : Sum  Inputs=-+|
  Sum1 : Sum  Inputs=+-|
  Terminator : Terminator
  Terminator1 : Terminator
  Angular acc des : Outport
  Control_in : Outport  Port=2
  wires:
  Lat_dir Dyn Inversion: beta_dot->r_c/1(r_c) -> Display6/1, Body Rates Controller/3(r_ref)
  Bus Selector3/1 -> Ref Model and P Controller/2  "<SS meas (rad)>"
  p des (rad/s)/1 -> Body Rates Controller/1(p_ref)
  Long Dyn Inversion: alpha_dot ->q/1(q_c) -> Display1/1, Body Rates Controller/2(q_ref)
  beta des (rad)/1 -> Ref Model and P Controller/1
  Longitudinal Controller: AoA or A_w_z/3(alpha_dot_c) -> Long Dyn Inversion: alpha_dot ->q/1(alpha_dot_c), Display/1
  AoA des (rad)/1 -> Longitudinal Controller: AoA or A_w_z/2(AoA des (rad))
  Anti-windup AoA/1 -> Longitudinal Controller: AoA or A_w_z/4(Anti-windup AoA)
  Anti-windup A_w_z/1 -> Longitudinal Controller: AoA or A_w_z/3(Anti-windup A_w_z)
  A_w_z des/1 -> Longitudinal Controller: AoA or A_w_z/1(A_w_z des)
  Sum/1 -> Display4/1, "Sigmoid "/1(In), Angular acc des/1  "v"
  Body Rates Controller/4(Angular acc des (rad/s^2)) -> Display3/1, Sum/2  "v_p+v_dot_ff"
  Bus Creator/1 -> On-line (adaptive) multi-layer NNs/3(NN variables)
  Memory/1 -> On-line (adaptive) multi-layer NNs/1(v_ad^ prev)
  Body Rates Controller/2(p_chanel vars) -> Bus Creator/2  "p_chanel_vars"
  Body Rates Controller/1(q_chanel vars) -> Bus Creator1/3  "q_chanel_vars"
  Longitudinal Controller: AoA or A_w_z/1(A_chanel vars) -> Bus Creator1/1  "A_chanel vars"
  Longitudinal Controller: AoA or A_w_z/2(alpha_chanel vars) -> Bus Creator1/2  "alpha_chanel vars"
  Bus Creator1/1 -> Bus Creator/1  "Long chanel"
  Ref Model and P Controller/2 -> Bus Creator2/1  "beta_sf_dot"
  Ref Model and P Controller/3 -> Sum1/1, Bus Creator2/2  "beta_sf"
  Sum1/1 -> Bus Creator2/3  "beta_err"
  Ref Model and P Controller/4 -> Sum1/2
  Ref Model and P Controller/5 -> Bus Creator2/4  "K_b_beta"
  Body Rates Controller/3(r_chanel vars) -> Bus Creator3/1  "r_chanel vars"
  Bus Creator2/1 -> Bus Creator3/2  "beta_chanel vars"
  Bus Creator3/1 -> Bus Creator/3  "beta_r_chanel"
  Anti-windup beta/1 -> Terminator1/1
  "Sigmoid "/1(Out) -> Memory/1
  On-line (adaptive) multi-layer NNs/1(v_ad^) -> Sum/1, Display2/1  "v_ad^"
  Ref Model and P Controller/1 -> Display5/1, Lat_dir Dyn Inversion: beta_dot->r_c/1(beta_dot_c)
  All measures/1 -> On-line (adaptive) multi-layer NNs/2(All_meas), Body Rates Controller/4(All_meas), Lat_dir Dyn Inversion: beta_dot->r_c/2(All_meas), Bus Selector3/1, Long Dyn Inversion: alpha_dot ->q/2(All_meas), Longitudinal Controller: AoA or A_w_z/5(All meas)
  Anti-windup signals/1 -> Terminator/1
  Ground/1 -> Control_in/1

== system F16ASYM_Controlled_ACC/Primary Controller/PI Primary Controller ==
  A_w_z des : Inport
  AoA des (rad) : Inport  Port=2
  p des (rad/s) : Inport  Port=3
  beta des (rad) : Inport  Port=4
  Anti-windup A_w_z : Inport  Port=5
  Anti-windup AoA : Inport  Port=6
  Anti-windup beta : Inport  Port=7
  All measures : Inport  Port=8
  Anti-windup signals : Inport  Port=9
  Body Rates Controller : Subsystem
  Bus Selector3 : BusSelector  OutputSignals=signal1.SS meas (rad)
  Display{,1..3} (4 alike) : Display
  Ground : Ground
  Lat_dir Dyn Inversion: beta_dot->r_c : Subsystem
  Long Dyn Inversion: alpha_dot ->q : Subsystem
  Longitudinal Controller: AoA or A_w_z : Subsystem  Variant=on  OverrideUsingVariant=Controller of A_w_z
  PI Controller: beta  controller : Adaptive_FaultTolerantControl/PI Controller  delta=0  K_a=0  y_i=trim_state(9)  Des_way=auto  omega_n=2  xi=1  Z1=-50  K_b=6  f_i=0.25  f_c=1
  Angular acc des : Outport
  Control_in : Outport  Port=2
  wires:
  A_w_z des/1 -> Longitudinal Controller: AoA or A_w_z/1(A_w_z des)
  Anti-windup A_w_z/1 -> Longitudinal Controller: AoA or A_w_z/3(Anti-windup A_w_z)
  Anti-windup AoA/1 -> Longitudinal Controller: AoA or A_w_z/4(Anti-windup AoA)
  AoA des (rad)/1 -> Longitudinal Controller: AoA or A_w_z/2(AoA des (rad))
  Longitudinal Controller: AoA or A_w_z/1(alpha_dot_c) -> Display/1, Long Dyn Inversion: alpha_dot ->q/1(alpha_dot_c)
  All measures/1 -> Bus Selector3/1, Lat_dir Dyn Inversion: beta_dot->r_c/2(All_meas), Body Rates Controller/4(All_meas), Longitudinal Controller: AoA or A_w_z/5(All meas), Long Dyn Inversion: alpha_dot ->q/2(All_meas)
  Anti-windup beta/1 -> PI Controller: beta  controller/3
  beta des (rad)/1 -> PI Controller: beta  controller/1
  Long Dyn Inversion: alpha_dot ->q/1(q_c) -> Body Rates Controller/2(q_ref), Display1/1
  p des (rad/s)/1 -> Body Rates Controller/1(p_ref)
  Body Rates Controller/1(Angular acc des (rad/s^2)) -> Angular acc des/1
  PI Controller: beta  controller/1 -> Lat_dir Dyn Inversion: beta_dot->r_c/1(beta_dot_c), Display3/1
  Anti-windup signals/1 -> Body Rates Controller/5(All Anti-windup signals)
  Bus Selector3/1 -> PI Controller: beta  controller/2  "<SS meas (rad)>"
  Lat_dir Dyn Inversion: beta_dot->r_c/1(r_c) -> Body Rates Controller/3(r_ref), Display2/1
  Ground/1 -> Control_in/1

== system F16ASYM_Controlled_ACC/SI and FDI/SI and FDI: Realistic ==
  note: RECONFIGURATION PARAMETERS
      |
      | 24. mass  Estimated mass
      | 25. S_current_L
      | 26. S_current_R
      | 27. S_fin_current
      | 28. x_cg
      | 29. Jy
      | 30. Jxz
      | 31. Jz
      | 32. Jx
      | 33. EFF_el_L
      | 34. EFF_el_R
      | 35. EFF_ail_L
      | 36. EFF_ail_R
      | 37. EFF_rud
      | 38. EFF_lef_L
      | 39. EFF_lef_R
      | 40. Delta_C_Lift_X
      | 41. Delta_C_Drag_X
      | 42. Delta_C_m_X
  Inexistent Reconfig bus : Inport
  Control comms : Inport  Port=2
  All  meas : Inport  Port=3
  Bus Creator : BusCreator  Inputs=3
  FDI: Assumed? : Subsystem  VariantObject=FDI: Realsitic
  Mass props : Selector  InputPortWidth=6  IndexOptions=Index vector (dialog)  Indices=2:6  OutputSizes=1
  Mux : Mux  Inputs=[9 7 3]
  Mux1 : Mux  Inputs=3
  SI : Subsystem
  mass : Selector  InputPortWidth=6  IndexOptions=Index vector (dialog)  Indices=1  OutputSizes=1
  Est reconf params : Outport
  wires:
  All  meas/1 -> FDI: Assumed?/2(All  meas), SI/2(All meas)
  FDI: Assumed?/3(Effectiveness) -> SI/1(Control Eff), Mux/2
  Mux/1 -> Bus Creator/3  "Reconfig signal"
  FDI: Assumed?/2(Blockades now) -> Bus Creator/2
  FDI: Assumed?/1(Blockades at) -> Bus Creator/1
  Bus Creator/1 -> Est reconf params/1
  Inexistent Reconfig bus/1 -> FDI: Assumed?/1(Inexistent Reconfig bus)
  Control comms/1 -> SI/3(Control comms)
  mass/1 -> Mux1/1
  SI/2(Est Surfs) -> Mux1/2
  Mass props/1 -> Mux1/3
  SI/1(Est Mass props) -> Mass props/1, mass/1
  Mux1/1 -> Mux/1
  SI/3(Est Aero changes) -> Mux/3

== system F16ASYM_Controlled_ACC/SI and FDI/SI and FDI: Unrealistic ==
  Inexistent Reconfig bus : Inport
  Control comms : Inport  Port=2
  All  meas : Inport  Port=3
  Terminator : Terminator
  Terminator1 : Terminator
  Est reconf params : Outport
  wires:
  Inexistent Reconfig bus/1 -> Est reconf params/1
  All  meas/1 -> Terminator/1
  Control comms/1 -> Terminator1/1

== system F16ASYM_Controlled_ACC/Speed-Throttle control/Stall protection TAS ==
  note: Margin here?
  TAS comm : Inport
  All meas : Inport  Port=2
  Bus Selector : BusSelector  OutputSignals=signal1.Alt meas (m),signal2.a
  Display : Display
  Gain2 : Gain  Gain=1.2
  Min TAS : Product  Inputs=**
  MinMax : MinMax  Function=max  Inputs=2
  Stall curve 1g : Lookup_n-D  NumberOfTableDimensions=1  BreakpointsForDimension1=Stall_curve.H_2  Table=Stall_curve.M_2  RemoveProtectionInput=on  RndMeth=Simplest  InputSameDT=on
  TAS des : Outport
  tag scope: Min_Mach=global
  wires:
  MinMax/1 -> TAS des/1
  TAS comm/1 -> MinMax/2
  All meas/1 -> Bus Selector/1
  Bus Selector/1 -> Stall curve 1g/1  "<Alt meas (m)>"
  Stall curve 1g/1 -> [Min_Mach], Min TAS/1  "Min M"
  Bus Selector/2 -> Min TAS/2  "<a>"
  Min TAS/1 -> Gain2/1
  Gain2/1 -> Display/1, MinMax/1
